simulink model "P1"  (R2023a)
settings: Solver=VariableStepAuto  StartTime=0.0  StopTime=10.0  MaxStep=0.001  RelTol=1e-3
values from neighbouring files (symbols this model uses):
  g = 9.81    [parametrosP1.m]
  l1 = 0.3    [parametrosP1.m]
  l2 = 0.25    [parametrosP1.m]
  m1 = 0.2    [parametrosP1.m]
  m2 = 0.1    [parametrosP1.m]
settings Model: Creator=aquet  LastModifiedBy=aquet

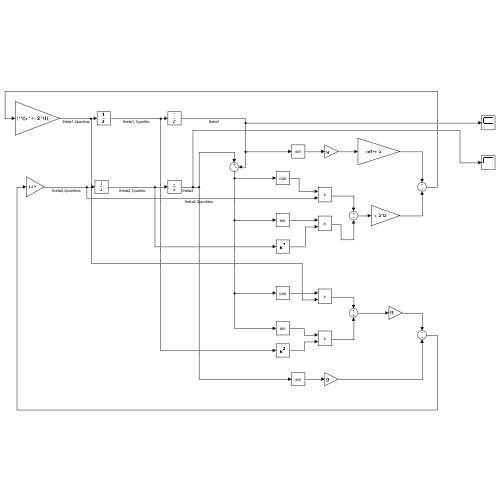
[thumbnail: Simulink's stored preview of the top-level diagram]
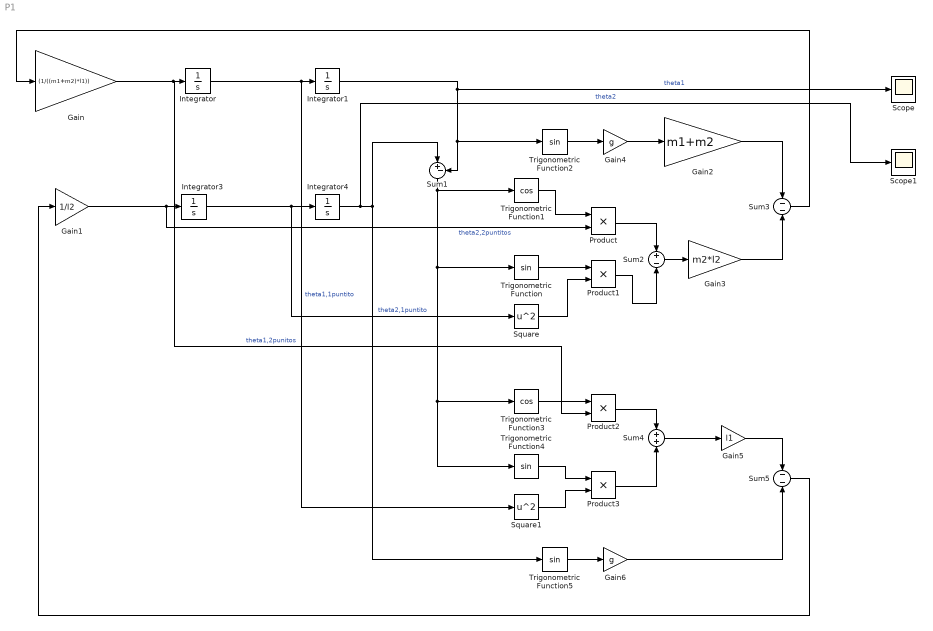
== system P1 ==
  Gain : Gain  Gain=(1/((m1+m2)*l1))
  Gain1 : Gain  Gain=1/l2
  Gain2 : Gain  Gain=m1+m2
  Gain3 : Gain  Gain=m2*l2
  Gain4 : Gain  Gain=g
  Gain5 : Gain  Gain=l1
  Gain6 : Gain  Gain=g
  Integrator : Integrator
  Integrator1 : Integrator
  Integrator3 : Integrator
  Integrator4 : Integrator  InitialCondition=(35*pi)/180
  Product{,1..3} (4 alike) : Product
  Scope : Scope
  Scope1 : Scope
  Square : Math  Operator=square
  Square1 : Math  Operator=square
  Sum1 : Sum  Inputs=|+-
  Sum2 : Sum  Inputs=+-
  Sum3 : Sum  Inputs=--
  Sum4 : Sum
  Sum5 : Sum  Inputs=--
  Trigonometric Function{,2,4..5} (4 alike) : Trigonometry
  Trigonometric Function1 : Trigonometry  Operator=cos
  Trigonometric Function3 : Trigonometry  Operator=cos
  wires:
  Gain/1 -> Integrator/1, Product2/2  "theta1,2punitos"
  Integrator/1 -> Square1/1, Integrator1/1  "theta1,1puntito"
  Integrator1/1 -> Scope/1, Sum1/2, Trigonometric Function2/1  "theta1"
  Gain1/1 -> Product/2, Integrator3/1  "theta2,2puntitos"
  Integrator3/1 -> Square/1, Integrator4/1  "theta2,1puntito"
  Integrator4/1 -> Scope1/1, Sum1/1, Trigonometric Function5/1  "theta2"
  Trigonometric Function1/1 -> Product/1
  Sum1/1 -> Trigonometric Function4/1, Trigonometric Function3/1, Trigonometric Function/1, Trigonometric Function1/1
  Trigonometric Function/1 -> Product1/1
  Square/1 -> Product1/2
  Product/1 -> Sum2/1
  Product1/1 -> Sum2/2
  Trigonometric Function2/1 -> Gain4/1
  Sum2/1 -> Gain3/1
  Gain4/1 -> Gain2/1
  Gain3/1 -> Sum3/2
  Gain2/1 -> Sum3/1
  Sum3/1 -> Gain/1
  Trigonometric Function3/1 -> Product2/1
  Trigonometric Function4/1 -> Product3/1
  Square1/1 -> Product3/2
  Product2/1 -> Sum4/1
  Product3/1 -> Sum4/2
  Gain5/1 -> Sum5/1
  Sum4/1 -> Gain5/1
  Trigonometric Function5/1 -> Gain6/1
  Gain6/1 -> Sum5/2
  Sum5/1 -> Gain1/1
